simulink model "mass_sim"  (R2015a)
settings: Solver=ode45  StartTime=0.0  StopTime=10000  RelTol=1e-3
InitFcn:
  | param
undefined symbols (not defined in the file or in its folder): drawMSD
libraries: simulink x1
settings Model: Creator=beard  LastModifiedBy=beard
settings DataIOCC: SignalLoggingSaveFormat=ModelDataLogs
settings OptimizationCC: ExpressionDepthLimit=2147483647  InitFltsAndDblsToZero=on
settings DebuggingCC: UnderspecifiedInitializationDetection=Classic  MergeDetectMultiDrivingBlocksExec=none  SolverPrmCheckMsg=warning  FcnCallInpInsideContextMsg=UseLocalSettings  StateNameClashWarn=warning  StrictBusMsg=Warning
settings GRTTargetCC: CombineOutputUpdateFcns=off  GRTInterface=on

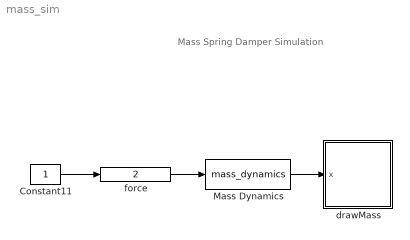
== system mass_sim ==
  note: Mass Spring Damper Simulation
  Constant11 : Constant
  Mass Dynamics : S-Function  FunctionName=mass_dynamics  Parameters=AP
  drawMass : Subsystem
      mask init:
      | % drawing parameters
      | L = 5;
      | w = 1;
      mask Display: image(imread('tv.jpg'))
  force : simulink/Math Operations/Slider Gain  low=-10  gain=2  high=10
  wires:
  Constant11/1 -> force/1
  Mass Dynamics/1 -> drawMass/1(x)
  force/1 -> Mass Dynamics/1

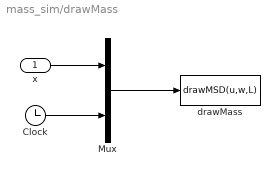
== system mass_sim/drawMass ==
  x : Inport
  Clock : Clock
  Mux : Mux  Inputs=2
  drawMass : MATLABFcn  MATLABFcn=drawMSD(u,w,L)  OutputDimensions=0  SampleTime=0.1
  wires:
  Clock/1 -> Mux/2
  x/1 -> Mux/1
  Mux/1 -> drawMass/1
